simulink model "AD9625"  (R2019b)
settings: Solver=FixedStepDiscrete  StartTime=0.0  StopTime=0.00002  FixedStep=1/2500e6  RelTol=1e-3  EnableMultiTasking=on
settings Model: Creator=tmacleod  LastModifiedBy=ian
settings SolverCC: AutoInsertRateTranBlk=on
settings DataIOCC: LimitDataPoints=on  SaveFormat=Array  ReturnWorkspaceOutputs=off
settings OptimizationCC: LifeSpan=inf
settings DebuggingCC: SolverPrmCheckMsg=warning  SFUnexpectedBacktrackingDiag=warning  SFNoUnconditionalDefaultTransitionDiag=warning  SFExecutionAtInitializationDiag=none  ArithmeticOperatorsInVariantConditions=warning
settings HardwareCC: ProdBitPerPointer=32  ProdBitPerSizeT=32  ProdBitPerPtrDiffT=32  ProdLargestAtomicFloat=None  ProdIntDivRoundTo=Undefined  ProdEndianess=Unspecified  ProdWordSize=32  ProdHWDeviceType=32-bit Generic
settings ModelReferenceCC: PropagateSignalLabelsOutOfModel=off
settings SFSimCC: SimUseLocalCustomCode=off  CustomCodeUndefinedFunction=UseInterfaceOnly
settings RTWCC: RTWUseLocalCustomCode=off
settings CodeAppCC: StateflowObjectComments=on
settings GRTTargetCC: TargetLangStandard=C89/C90 (ANSI)  GeneratePreprocessorConditionals=Disable all
settings ConfigComp: CovMetricSettings=dw  CovHtmlReporting=on  CovSaveCumulativeToWorkspaceVar=on  CovSaveSingleToWorkspaceVar=on  CovExternalEMLEnable=off  CovSFcnEnable=off

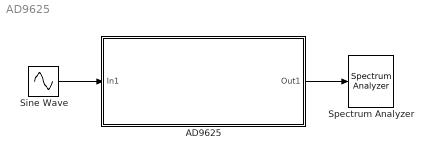
== system AD9625 ==
  AD9625 : Subsystem  mask{maskMode=ADC Only, maskDecimation=8, maskGain=0, maskNcoFreq=100e6, maskFclk=2500e6, maskTessitura=147e6, maskExtJitter=60e-15, maskInputConfig=Normalized}
      mask prompts: maskMode "Mode of Operation"; maskDecimation "DDC Decimation"; maskGain "DDC Gain (dB)"; maskNcoFreq "NCO Frequency (Hz)"; maskFclk "Sampling Clock Frequency (Hz)"; maskTessitura "Mean Frequency (Hz)"; maskExtJitter "RMS Clock Jitter"; maskInputConfig "Input Configuration"
      mask init:
      | set_param([gcb '/AD9625 System Object'], 'Mode', maskMode);
      | set_param([gcb '/AD9625 System Object'], 'Decimation', maskDecimation);
      | set_param([gcb '/AD9625 System Object'], 'Gain', maskGain);
      | set_param([gcb '/AD9625 System Object'], 'NcoFreq', maskNcoFreq);
      | set_param([gcb '/AD9625 System Object'], 'Fclk', maskFclk);
      | set_param([gcb '/AD9625 System Object'], 'Tessitura', maskTessitura);
      | set_param([gcb '/AD9625 System Object'], 'ExtJitter', maskExtJitter);
      | set_param([gcb '/AD9625 System Object'], 'InputConfig', maskInputConfig);
      mask TypeOptions maskMode: ADC Only | ADC + DDC
      mask Callback maskMode:
      | % Get the mask parameter values. This is a cell
      | %   array of strings.
      | maskStr = get_param(gcb,'maskMode');
      | 
      | % The pop-up menu is the first mask parameter.
      | %   Check the value selected in the pop-up
      | if strcmp(maskStr,'ADC Only'),
      | 
      |     % Set the visibility of both parameters on when
      |     %   User-defined is selected in the pop-up.
      | 
      |     set_param(gcb,'MaskVisibilities',{'on';'off';'off';'off';'on';'on';'on';'on'}),
      | 
      | else
      | 
      |     % Turn off the visibility of the Value field
      |     %   when User-defined is not selected.
      | 
      |     set_param(gcb,'MaskVisibilities',{'on';'on';'on';'on';'on';'on';'on';'on'}),
      | 
      |     % Set the string in the Values field equal to the
      |     % string selected in the Gain pop-up menu.
      | 
      |     %maskStr{2}=maskStr{1};
      |     %set_param(gcb,'editvalue',maskStr);
      | end
      mask TypeOptions maskDecimation: 8 | 16
      mask TypeOptions maskGain: 0 | 6 | 12 | 18
      mask TypeOptions maskInputConfig: Normalized | Absolute
      mask Display:
      | port_label('input', 1, 'in (V)')
      | port_label('output', 1, 'out (Codes)')
  Sine Wave : Sin  Amplitude=0.89  Frequency=2*pi*147e6  SampleTime=0
  Spectrum Analyzer : SpectrumAnalyzer
  wires:
  AD9625/1(Out1) -> Spectrum Analyzer/1
  Sine Wave/1 -> AD9625/1(In1)

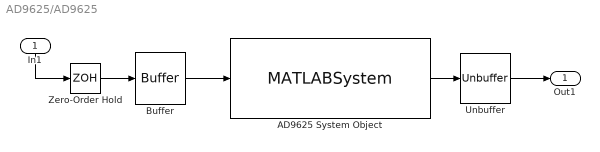
== system AD9625/AD9625 ==
  In1 : Inport
  AD9625 System Object : MATLABSystem  System=AD9625_sysobj  Mode=ADC Only  Gain=0  NcoFreq=100e6  Fclk=2500e6  Tessitura=147e6  ExtJitter=60e-15  InputConfig=Normalized  SimulateUsing=Interpreted execution
      settings: Decimation=8
      mask Type: AD9625_sysobj
      mask Display:
      | disp('AD9625');
      | port_label('input',1,'in (V)');
      | port_label('output',1,'out (Code)');
  Buffer : Buffer
  Unbuffer : Unbuffer
  Zero-Order Hold : ZeroOrderHold  SampleTime=1/2500e6
  Out1 : Outport
  wires:
  AD9625 System Object/1 -> Unbuffer/1
  In1/1 -> Zero-Order Hold/1
  Buffer/1 -> AD9625 System Object/1
  Zero-Order Hold/1 -> Buffer/1
  Unbuffer/1 -> Out1/1
